simulink model "RC_RC"  (R2013a)
settings: Solver=ode3  SolverMode=SingleTasking  StartTime=0.0  StopTime=19e-3  FixedStep=FS/50  MaxStep=1e-4  RelTol=1e-3
InitFcn:
  | %%%%%%  set scope time range
  | T_STOP=str2num(get_param(gcs,'StopTime'));
  | if numel(T_STOP) > 1
  |    T_STOP=T_STOP(2);
  | else
  |    T_STOP=T_STOP(1);
  | end
  | T_STOP=num2str(T_STOP);
  | 
  | %%%%%%  set scope time range in system @init_callback_fct
  | T_STOP=num2str(str2num(get_param(gcs,'StopTime')));
  | 
  | childs = allchild(0);
  | sol=strfind(upper(get(allchild(0),'Tag')),'VIEWER_PARAMETERS');
  | 
  | if iscell(sol)
  |    ind=find(~cellfun(@isempty, strfind(upper(get(allchild(0),'Tag')),'VIEWER_PARAMETERS')));
  | else
  |    ind=sol;
  | end
  | %ind=find(~cellfun(@isempty, {strfind(upper(get(allchild(0),'Tag')),'VIEWER_PARAMETERS'),[]}))
  | if ~isempty(ind)
  |    for k=1:length(childs(ind))
  |       set_param(getfield(get(childs(ind(k)),'UserData'),'block'),'TimeRange',T_STOP);
  |       get_param(getfield(get(childs(ind(k)),'UserData'),'block'),'TimeRange');
  | %    set_param(getfield(get(childs(ind),'UserData'),'block'),'TimeRange',T_STOP);
  | %    get_param(getfield(get(childs(ind),'UserData'),'block'),'TimeRange');
  |    end
  | else
  |     warning(sprintf('VIEWER_PARAMETERS object not found\nOpen the config dialog by hand for the first sim start'))
  | end
values from neighbouring files (symbols this model uses):
  Aw = 1.2    [GalvoModel_v6_sys.m]
  FS = 5e-6    (= 5e-06)    [GalvoModel_v4_sys.m]    (also in GalvoModel_v6_sys.m = 5e-05; Galvo_process_analyze.m = 0.0001)
  T1 = R1*C1    (= 0.000264)    [GalvoModel_v6_sys.m]
libraries: simulink x1
settings Model: BufferReuse=off  Creator=mainster  LastModifiedBy=mainster
settings SolverCC: AutoInsertRateTranBlk=on
settings OptimizationCC: InlineParams=on  BufferReuse=off
settings DebuggingCC: InitInArrayFormatMsg=none
settings HardwareCC: ProdLargestAtomicInteger=Long  ProdLargestAtomicFloat=Double  ProdEndianess=LittleEndian  ProdHWDeviceType=ARM Compatible->ARM Cortex

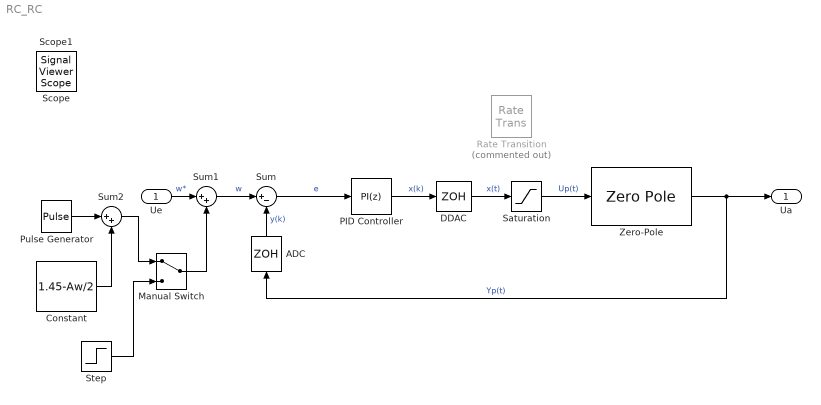
== system RC_RC ==
  Ue : Inport  SampleTime=FS
  ADC : ZeroOrderHold  SampleTime=FS
  Constant : Constant  Value=1.45-Aw/2
  DDAC : ZeroOrderHold  SampleTime=FS
  Manual Switch : ManualSwitch  SampleTime=FS
  PID Controller : simulink/Continuous/PID Controller  Controller=PI  TimeDomain=Discrete-time  SampleTime=FS  IntegratorMethod=Forward Euler  FilterMethod=Forward Euler  Form=Parallel  P=1.84546966370507  I=3745.38790742202  D=9.0248898483108e-05  N=10930.7783722874  InitialConditionSource=internal  InitialConditionForIntegrator=0  InitialConditionForFilter=0  ExternalReset=none  LimitOutput=off  UpperSaturationLimit=inf  LowerSaturationLimit=-inf  LinearizeAsGain=on  AntiWindupMode=none  Kb=1  TrackingMode=off  Kt=1  PParamMin=[]  PParamMax=[]  IParamMin=[]  IParamMax=[]  DParamMin=[]  DParamMax=[]  NParamMin=[]  NParamMax=[]  KbParamMin=[]  KbParamMax=[]  KtParamMin=[]  KtParamMax=[]  POutMin=[]  POutMax=[]  IOutMin=[]  IOutMax=[]  DOutMin=[]  DOutMax=[]  NOutMin=[]  NOutMax=[]  KbOutMin=[]  KbOutMax=[]  KtOutMin=[]  KtOutMax=[]  IntegratorOutMin=[]  IntegratorOutMax=[]  FilterOutMin=[]  FilterOutMax=[]  SumOutMin=[]  SumOutMax=[]  SumI1OutMin=[]  SumI1OutMax=[]  SumI2OutMin=[]  SumI2OutMax=[]  SumI3OutMin=[]  SumI3OutMax=[]  SumDOutMin=[]  SumDOutMax=[]  SaturationOutMin=[]  SaturationOutMax=[]  IntegratorContinuousStateAttributes=''  IntegratorStateMustResolveToSignalObject=off  IntegratorRTWStateStorageClass=Auto  FilterContinuousStateAttributes=''  FilterStateMustResolveToSignalObject=off  FilterRTWStateStorageClass=Auto
      settings: AttributesFormatString=Kp: %<P>\nKi: %<I>\nKd: %<D>\nN: %<N>
  Pulse Generator : DiscretePulseGenerator  PulseType=Time based  Amplitude=Aw  Period=1/200  PulseWidth=50  PhaseDelay=0.5e-3  SampleTime=FS
  Rate Transition : RateTransition  Commented=on  OutPortSampleTime=FS
  Saturation : Saturate  UpperLimit=2.85  LowerLimit=0
      settings: AttributesFormatString=Up_lim=%<UpperLimit>\nLo_lim=%<LowerLimit>
  Step : Step  Time=1e-3  SampleTime=FS
      settings: AttributesFormatString=Time:%<Time>\nAmp:%<After>
  Sum : Sum  Inputs=|+-  SampleTime=FS
  Sum1 : Sum  Inputs=|++  SampleTime=FS
  Sum2 : Sum  Inputs=|++  SampleTime=FS
  Zero-Pole : ZeroPole  Zeros=[]  Poles=[-1/T1 -1/T1]  Gain=(1/T1)^2
  Ua : Outport  SampleTime=FS
  Scope : SignalViewerScope  IOType=viewer  NumInputPorts=3  ZoomMode=xonly  LegendLocations=|  RefreshTime=0.035000
      | 0.75993     0.90863     0.18653    0.043765
      | 0.77318     0.61579     0.17329     0.02457
      | 0.75993     0.28332     0.18653    0.043765
      settings: ShowLegends=on  TimeRange=0.019  YMin=0~-1~0  YMax=2.5~5~2.5
  Scope1 : SignalViewerScope  IOType=viewer  ZoomMode=xonly  RefreshTime=0.035000
      settings: ShowLegends=on  TimeRange=0.019  YMin=-1  YMax=3
  wires:
  Sum/1 -> PID Controller/1  "e"
  Sum1/1 -> Sum/1  "w"
  Ue/1 -> Sum1/1  "w*"
  Zero-Pole/1 -> Ua/1, ADC/1  "Yp(t)"
  PID Controller/1 -> DDAC/1  "x(k)"
  ADC/1 -> Sum/2  "y(k)"
  DDAC/1 -> Saturation/1  "x(t)"
  Step/1 -> Manual Switch/2
  Manual Switch/1 -> Sum1/2
  Sum2/1 -> Manual Switch/1
  Pulse Generator/1 -> Sum2/1
  Constant/1 -> Sum2/2
  Saturation/1 -> Zero-Pole/1  "Up(t)"
